simulink model "DC_motor"  (R2023a)
settings: Solver=VariableStepAuto  StartTime=0.0  StopTime=10.0  RelTol=1e-3
values from neighbouring files (symbols this model uses):
  C_M = 1.3    [constants.m]
  J_motor = 7*10^-6    (= 7e-06)    [constants.m]
  L_anch = 15 * 10^-4    (= 0.0015)    [constants.m]
  L_ov = 0.013    [constants.m]
  R_anch = 8    [constants.m]
settings Model: Creator=windowskonon  LastModifiedBy=windowskonon

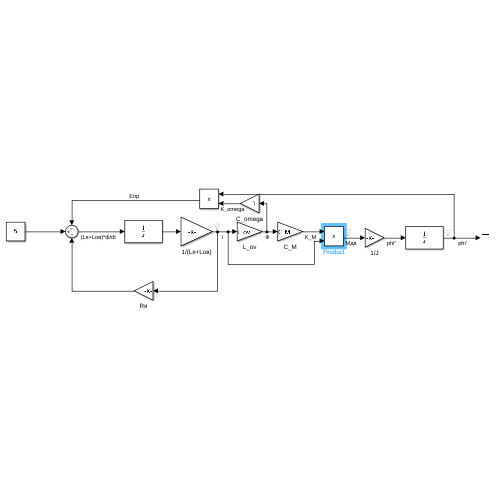
[thumbnail: Simulink's stored preview of the top-level diagram]
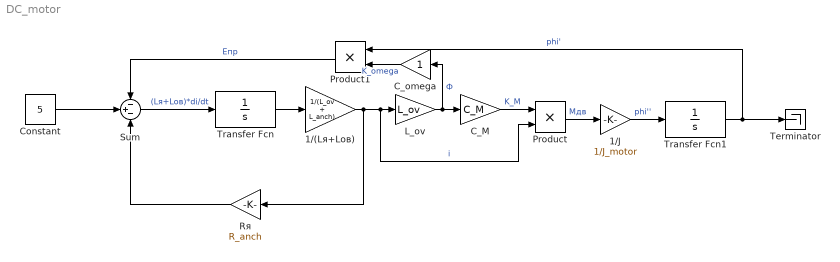
== system DC_motor ==
  1/(Lя+Lов) : Gain  Gain=1/(L_ov + L_anch)
  1/J : Gain  Gain=1/J_motor
  C_M : Gain  Gain=C_M
  C_omega : Gain
  Constant : Constant  Value=5
  L_ov : Gain  Gain=L_ov
  Product : Product
  Product1 : Product
  Rя : Gain  Gain=R_anch
  Sum : Sum  Inputs=-+-
  Terminator : Terminator
  Transfer Fcn : TransferFcn  Denominator=[1 0]
  Transfer Fcn1 : TransferFcn  Denominator=[1 0]
  wires:
  Sum/1 -> Transfer Fcn/1  "(Lя+Lов)*di/dt"
  Transfer Fcn/1 -> 1/(Lя+Lов)/1
  1/(Lя+Lов)/1 -> Rя/1, Product/2, L_ov/1  "i"
  L_ov/1 -> C_omega/1, C_M/1  "Ф"
  C_M/1 -> Product/1  "K_M"
  Product/1 -> 1/J/1  "Mдв"
  1/J/1 -> Transfer Fcn1/1  "phi''"
  Transfer Fcn1/1 -> Product1/1, Terminator/1  "phi'"
  Rя/1 -> Sum/3
  C_omega/1 -> Product1/2  "K_omega"
  Product1/1 -> Sum/1  "Eпр"
  Constant/1 -> Sum/2
